simulink model "DTNS_SIM"  (R2022a)
settings: Solver=ode4  StartTime=0.0  StopTime=100  FixedStep=0.01  RelTol=1e-3
PreLoadFcn:
  | listing = dir;
  | if (contains([listing.name], 'MAP')) &&  (contains([listing.name], 'DTNS_SIM.slx'))
  |     addpath('./AGR', './TRN', './TCAF', './FTG', './DYN', './FLCC', './GPS', './RALT', './INS', './MAP');
  |     addpath('./MAP/MAP_DB');
  | else
  |     warning('[DTNS_SIM.slx]는 DTNS 프로젝트 최상단 경로에 위치해야 합니다.');
  | end
  | 
  | load('BUS_STRUCTURE_DYN.mat');
  | load('BUS_STRUCTURE_FLCC.mat');
  | load('BUS_STRUCTURE_RALT.mat');
  | load('BUS_STRUCTURE_INS.mat');
  | load('BUS_STRUCTURE_GPS.mat');
  | load('BusStructureTRN.mat');
  | load('BusStructureLOSR.mat');
  | load('BusStructureHR.mat');
  | load('BusStructureCR.mat');
  | FTG_initState;
InitFcn:
  | listing = dir;
  | if (contains([listing.name], 'MAP')) &&  (contains([listing.name], 'DTNS_SIM.slx'))
  |     addpath('./AGR', './TRN', './TCAF', './FTG', './DYN', './FLCC', './GPS', './RALT', './INS', './MAP');
  |     addpath('./MAP/MAP_DB');
  | else
  |     warning('[DTNS_SIM.slx]는 DTNS 프로젝트 최상단 경로에 위치해야 합니다.');
  | end
  | 
  | load('BUS_STRUCTURE_DYN.mat');
  | load('BUS_STRUCTURE_FLCC.mat');
  | load('BUS_STRUCTURE_RALT.mat');
  | load('BUS_STRUCTURE_INS.mat');
  | load('BUS_STRUCTURE_GPS.mat');
  | load('BusStructureTRN.mat');
  | load('BusStructureLOSR.mat');
  | load('BusStructureHR.mat');
  | load('BusStructureCR.mat');
  | FTG_initState;
undefined symbols (not defined in the file or in its folder): initState
libraries: aerolibconvert2 x16, simulink_extras x5
(part 1 of 2)
settings Model: PacingRate=3  Creator=ASCL  LastModifiedBy=ASCL
settings SolverCC: PositivePriorityOrder=on  AutoInsertRateTranBlk=on
settings DataIOCC: ExternalInput=FTGScenario.getElement('IN_STICK'), [], [], FTGScenario.getElement('IN_FLIGHT_CMD'), []  LoadExternalInput=on  SaveOutput=off  DSMLogging=off  ReturnWorkspaceOutputs=off
settings OptimizationCC: BlockReduction=off  DefaultParameterBehavior=Inlined  UseDivisionForNetSlopeComputation=on  GainParamInheritBuiltInType=on  UseFloatMulNetSlope=on  ExpressionFolding=off  PassReuseOutputArgsAs=Individual arguments  ZeroExternalMemoryAtStartup=off  ZeroInternalMemoryAtStartup=off  EfficientFloat2IntCast=on  LifeSpan=inf  OptimizeBlockOrder=speed  DifferentSizesBufferReuse=on  EfficientTunableParamExpr=on
settings DebuggingCC: SignalInfNanChecking=warning  ReadBeforeWriteMsg=EnableAllAsError  WriteAfterWriteMsg=EnableAllAsError  WriteAfterReadMsg=EnableAllAsError  IntegerOverflowMsg=error  ParameterTunabilityLossMsg=error  UniqueDataStoreMsg=error  AssertControl=DisableAll  NonBusSignalsTreatedAsBus=error  SFInvalidInputDataAccessInChartInitDiag=error  SFTransitionOutsideNaturalParentDiag=error  SFUnreachableExecutionPathDiag=error  SFUndirectedBroadcastEventsDiag=error  IntegerSaturationMsg=error
settings HardwareCC: ProdBitPerPointer=32  ProdBitPerSizeT=32  ProdBitPerPtrDiffT=32  ProdLargestAtomicInteger=Long  ProdLargestAtomicFloat=Double  ProdEndianess=BigEndian  ProdWordSize=32  ProdLongLongMode=on  ProdHWDeviceType=Freescale->MPC83xx
settings ModelReferenceCC: ModelReferenceNumInstancesAllowed=Single
settings SFSimCC: SimCustomHeaderCode="#include \"MAP.h\""  SimUserSources=MAP.c  SimUserLibraries=WS2_32.LIB  CompileTimeRecursionLimit=0  EnableRuntimeRecursion=off  MATLABDynamicMemAlloc=off  CustomCodeGlobalsAsFunctionIO=on
settings RTWCC: SystemTargetFile=ert.tlc  TemplateMakefile=ert_default_tmf  GenerateReport=on  RTWUseSimCustomCode=on  CustomHeaderCode="#include \"MAP.h\""  CustomSource=MAP.c  CustomLibrary=WS2_32.LIB  BuildConfiguration=Faster Runs  IncludeHyperlinkInReport=on  LaunchReport=on  GenerateTraceInfo=on  GenerateTraceReport=on  GenerateTraceReportSl=on  GenerateTraceReportSf=on  GenerateTraceReportEml=on  GenerateCodeMetricsReport=on
settings CodeAppCC: ForceParamTrailComments=on  IgnoreCustomStorageClasses=off  OperatorAnnotations=on  SimulinkDataObjDesc=on  SFDataObjDesc=on  MATLABFcnDesc=on  InsertBlockDesc=on  StateflowObjectComments=on  MATLABSourceComments=on  EnableCustomComments=on  InlinedPrmAccess=Macros  ReqsInCode=on
settings ERTTargetCC: TargetLangStandard=C99 (ISO)  UtilityFuncGeneration=Shared location  GenerateSampleERTMain=on  CombineSignalStateStructs=on  SuppressErrorStatus=on  SupportNonFinite=off  SupportVariableSizeSignals=on  ParenthesesLevel=Standards  CastingMode=Standards  GenerateSharedConstants=off  InlinedParameterPlacement=NonHierarchical  ERTCustomFileTemplate=example_file_process.tlc  RateTransitionBlockCode=Function  PreserveIfCondition=on  ConvertIfToSwitch=off  EnableSignedLeftShifts=off  EnableSignedRightShifts=off

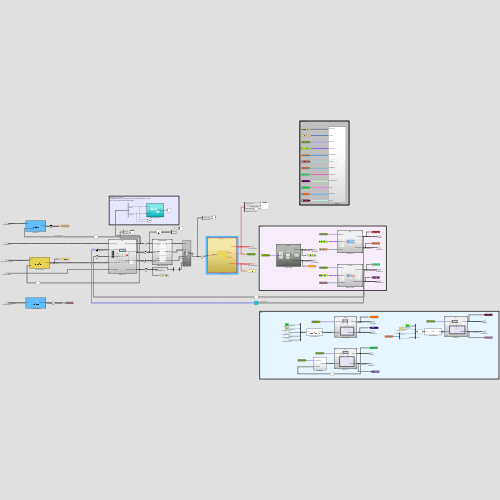
[thumbnail: Simulink's stored preview of the top-level diagram]
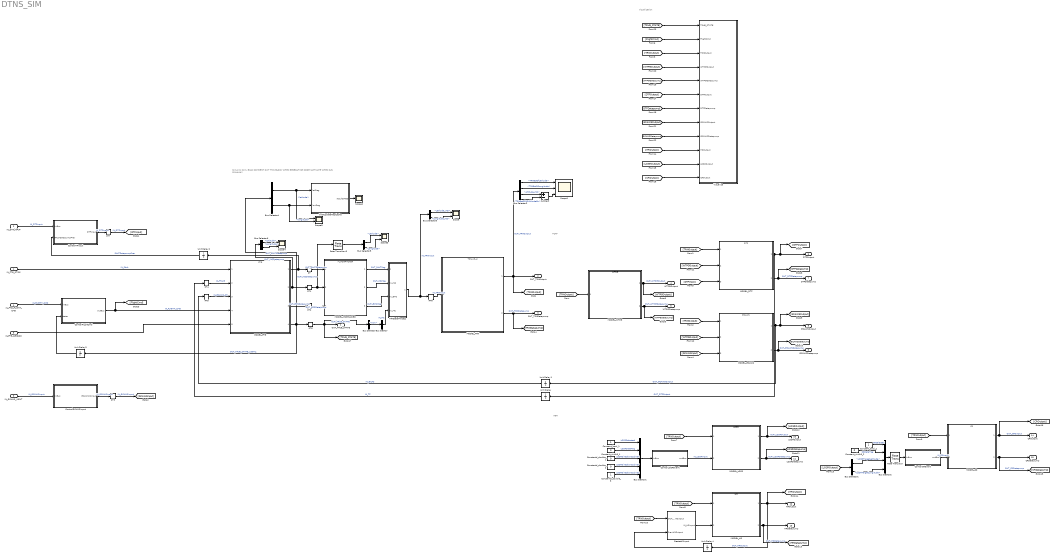
== system DTNS_SIM ==
  note: AGR
  note: TCAF
  note: Visualization
  note: Simulink Only Block
      | COMMENT OUT THIS BLOCK WHEN GENERATING CODE
      | (ACTIVATE WHEN RUN SIMULINK)
  IN_FTG_STICK : Inport  OutDataTypeStr=Bus: BUS_FLCC_STICK  SampleTime=0.01  Interpolate=off  BusOutputAsStruct=on
  IN_DTF_INPUT : Inport  Port=2  OutDataTypeStr=Bus: DTFInput  SampleTime=0.01  Interpolate=off  BusOutputAsStruct=on
  IN_GCAWS_INPUT : Inport  Port=3  OutDataTypeStr=Bus: GCAWSInput  SampleTime=0.01  Interpolate=off  BusOutputAsStruct=on
  IN_FTG_FLIGHT_CMD : Inport  Port=4  OutDataTypeStr=Bus: BUS_FLCC_FLIGHT_CMD  SampleTime=0.01  Interpolate=off  BusOutputAsStruct=on
  IN_FTG_SENSOR : Inport  Port=5  OutDataTypeStr=Bus: BUS_SENSOR_ALL_INPUTSTATUS  SampleTime=0.01  Interpolate=off  BusOutputAsStruct=on
  Bus Creator : BusCreator  Inputs=1  OutDataTypeStr=Bus: TRN_MC  NonVirtualBus=on
      settings: InheritFromInputs=off
  Bus Creator1 : BusCreator  Inputs=5  OutDataTypeStr=Bus: LOSRInput  NonVirtualBus=on
      settings: InheritFromInputs=off
  Bus Creator2 : BusCreator  Inputs=4  OutDataTypeStr=Bus: CRInput
      settings: InheritFromInputs=off
  Bus Selector : BusSelector  OutputSignals=wow
  Bus Selector1 : BusSelector  OutputSignals=LOSRTargetLatitude,LOSRTargetLongitude
  Bus Selector2 : BusSelector  OutputSignals=TRNEstOfLatitude,TRNEstOfLongitude,Altitude_INS,TRNEstOfINSAltitudeErr
  Bus Selector3 : BusSelector  OutputSignals=Latitude_INS,Longitude_INS
  Bus Selector4 : BusSelector  OutputSignals=latitude,longitude
  Bus Selector5 : BusSelector  OutputSignals=Latitude,Longitude
  Bus Selector6 : BusSelector  OutputSignals=Latitude,Longitude
  Constant_bool_1 : Constant  OutDataTypeStr=boolean  SampleTime=0.04
  Constant_bool_2 : Constant  OutDataTypeStr=boolean  SampleTime=0.04
  Constant_uint16_1 : Constant  Value=0  OutDataTypeStr=uint16  SampleTime=0.04
  Constant_uint16_2 : Constant  Value=0  OutDataTypeStr=uint16  SampleTime=0.04
  Constantd_double_1 : Constant  Value=0  OutDataTypeStr=double  SampleTime=0.04
  Constantd_double_2 : Constant  Value=0  OutDataTypeStr=double  SampleTime=0.04
  Constantd_double_3 : Constant  OutDataTypeStr=double  SampleTime=0.04
  ControlCREvent : MATLAB Function  TreatAsAtomicUnit=on  SystemSampleTime=0.04
  ControlFlightCmd : MATLAB Function  TreatAsAtomicUnit=on
  ControlGCAWSInput : MATLAB Function  TreatAsAtomicUnit=on
  ControlLOSREvent : MATLAB Function  TreatAsAtomicUnit=on  SystemSampleTime=0.04
  ControlTFInput : MATLAB Function  TreatAsAtomicUnit=on
  CreateHRInput : Subsystem  TreatAsAtomicUnit=on  PartitionName=CreateHRInput
      settings: RTWSystemCode=Nonreusable function
  InitNUpdateMapCache : Subsystem  TreatAsAtomicUnit=on  PartitionName=InitNUpdateMapCache
  MODEL_CR : ModelReference  ModelNameDialog=CR.slx  SimulationMode=Normal  ScheduleRatesWith=Schedule Editor  ModelReferenceVersion=1.263
  MODEL_DTF : ModelReference  ModelNameDialog=DTF.slx  SimulationMode=Normal  ScheduleRatesWith=Schedule Editor  ModelReferenceVersion=1.443
  MODEL_FTG : ModelReference  ModelNameDialog=FTG.slx  SimulationMode=Normal  ScheduleRatesWith=Schedule Editor  ModelReferenceVersion=1.714
  MODEL_GCAWS : ModelReference  ModelNameDialog=GCAWS.slx  SimulationMode=Normal  ScheduleRatesWith=Schedule Editor  ModelReferenceVersion=1.800
  MODEL_HR : ModelReference  ModelNameDialog=HR.slx  SimulationMode=Normal  ScheduleRatesWith=Schedule Editor  ModelReferenceVersion=1.389
  MODEL_LOSR : ModelReference  ModelNameDialog=LOSR.slx  SimulationMode=Normal  ScheduleRatesWith=Schedule Editor  ModelReferenceVersion=1.371
  MODEL_MSGPACKER : ModelReference  ModelNameDialog=M_MSGPACKER.slx  SimulationMode=Normal  ScheduleRatesWith=Schedule Editor  ModelReferenceVersion=1.319
  MODEL_TRN : ModelReference  ModelNameDialog=TRN_V3_2.slx  SimulationMode=Normal  ScheduleRatesWith=Schedule Editor  CachedPortDiscreteRates=[0.04]  ModelReferenceVersion=2.356
  MODEL_WTPG : ModelReference  ModelNameDialog=WTPG.slx  SimulationMode=Normal  ScheduleRatesWith=Schedule Editor  ModelReferenceVersion=1.459
  RT{,1..3,6..7} (6 alike) : RateTransition  OutPortSampleTime=0.04
  RT4 : RateTransition  OutPortSampleTime=0.01
  RT5 : RateTransition  OutPortSampleTime=0.01
  RT8 : RateTransition
  Rate Transition : RateTransition  OutPortSampleTime=0.04
  Rate Transition3 : RateTransition
  Scope{,3..5} (4 alike) : Scope  NumInputPorts=2
  Scope1 : Scope  NumInputPorts=3
  Scope2 : Scope
  Subtract : Sum  Inputs=+-
  TRNDataProcess : Subsystem  TreatAsAtomicUnit=on  PartitionName=TRNDataProcess
  Unit Delay{,1..2,4} (4 alike) : UnitDelay  SampleTime=-1  HasFrameUpgradeWarning=on
  Unit Delay3 : UnitDelay  InitialCondition=initState  SampleTime=0.01  HasFrameUpgradeWarning=on
  Visualize : Subsystem
  OUT_TRUE_STATE : Outport  OutDataTypeStr=Bus: BUS_DYN_STATE  BusOutputAsStruct=on
  OUT_TRNOutput : Outport  Port=2  OutDataTypeStr=Bus: TRNOutput
  OUT_TRNDatapump : Outport  Port=3  OutDataTypeStr=Bus: TRNDatapump
  WTPGOutput : Outport  Port=4  OutDataTypeStr=Bus: WTPGOutput
  WTPGDatapump : Outport  Port=5  OutDataTypeStr=Bus: WTPGDatapump
  DTFOutput : Outport  Port=6  OutDataTypeStr=Bus: DTFOutput
  DTFDatapump : Outport  Port=7  OutDataTypeStr=Bus: DTFDatapump
  GCAWSOutput : Outport  Port=8  OutDataTypeStr=Bus: GCAWSOutput
  GCAWSDatapump : Outport  Port=9  OutDataTypeStr=Bus: GCAWSDatapump
  LOSROutput : Outport  Port=10  OutDataTypeStr=Bus: LOSROutput  BusOutputAsStruct=on
  LOSRDatapump : Outport  Port=11  OutDataTypeStr=Bus: LOSRDatapump  BusOutputAsStruct=on
  HROutput : Outport  Port=12  OutDataTypeStr=Bus: HROutput  BusOutputAsStruct=on
  HRDatapump : Outport  Port=13  OutDataTypeStr=Bus: HRDatapump  BusOutputAsStruct=on
  CROutput : Outport  Port=14  OutDataTypeStr=Bus: CROutput  BusOutputAsStruct=on
  CRDatapump : Outport  Port=15  OutDataTypeStr=Bus: CRDatapump  BusOutputAsStruct=on
  wires:
  Bus Creator/1 -> TRNDataProcess/4(In_MC)  "IN_MC"
  MODEL_FTG/3 -> RT2/1  "OUT_GPSDatapump"
  MODEL_WTPG/2 -> [WTPGDatapump], WTPGDatapump/1  "OUT_WTPGDatapump"
  MODEL_GCAWS/2 -> [GCAWSDatapump], GCAWSDatapump/1  "OUT_GCAWSDatapump"
  MODEL_TRN/2 -> [TRNDatapump], OUT_TRNDatapump/1  "OUT_TRNDatapump"
  MODEL_GCAWS/1 -> GCAWSOutput/1, [GCAWSOutput], Unit Delay1/1  "OUT_GCAWSOutput"
  IN_GCAWS_INPUT/1 -> ControlGCAWSInput/1(inBus)  "IN_GCAWSInput"
  IN_FTG_FLIGHT_CMD/1 -> ControlFlightCmd/1(inBus)  "IN_FLIGHT_CMD"
  RT6/1 -> [TRUE_STATE], Bus Selector/1, OUT_TRUE_STATE/1  "OUT_TRUE_STATE"
  MODEL_FTG/2 -> Bus Selector6/1, RT1/1  "OUT_INSDatapump"
  Unit Delay1/1 -> RT5/1  "IN_GCAS"
  Unit Delay/1 -> RT4/1  "IN_TF"
  MODEL_FTG/1 -> RT/1, Unit Delay2/1  "OUT_RALTDatapump"
  IN_FTG_STICK/1 -> MODEL_FTG/1  "IN_Stick"
  MODEL_DTF/1 -> DTFOutput/1, [DTFOutput], Unit Delay/1  "OUT_DTFOutput"
  ControlFlightCmd/1(outBus) -> MODEL_FTG/4, [FlightCmd]  "IN_FLIGHT_CMD"
  IN_DTF_INPUT/1 -> ControlTFInput/1(inBus)  "IN_DTFInput"
  MODEL_MSGPACKER/3 -> TRNDataProcess/3(In_GPS)  "OUT_GPSMsg"
  MODEL_MSGPACKER/1 -> TRNDataProcess/1(In_RALT)  "OUT_RALTMsg"
  MODEL_MSGPACKER/2 -> TRNDataProcess/2(In_INS)  "OUT_INSMsg"
  InitNUpdateMapCache/1(resultDTED) -> Scope2/1
  IN_FTG_SENSOR/1 -> MODEL_FTG/5
  RT7/1 -> [DTFInput]  "IN_DTFInput"
  Unit Delay2/1 -> ControlTFInput/2(RALTDatapumpPrev)  "RALTDatapumpPrev"
  RT3/1 -> [GCAWSInput]  "IN_GCAWSInput"
  Unit Delay3/1 -> ControlFlightCmd/2(state)
  TRNDataProcess/1(TRN INPUT) -> Bus Selector3/1, RT8/1  "IN_TRNInput"
  RT/1 -> MODEL_MSGPACKER/1  "OUT_RALTDatapump"
  RT1/1 -> Rate Transition3/1, MODEL_MSGPACKER/2  "OUT_INSDatapump"
  RT2/1 -> MODEL_MSGPACKER/3  "OUT_GPSDatapump"
  RT4/1 -> MODEL_FTG/2  "IN_TF_25"
  RT5/1 -> MODEL_FTG/3  "IN_GCAWS_25"
  MODEL_FTG/4 -> Unit Delay3/1, Bus Selector4/1, RT6/1  "OUT_TRUE_STATE_100HZ"
  Constant_uint16_2/1 -> Bus Creator2/2  "CRDataTag"
  MODEL_HR/2 -> HRDatapump/1, [HRDatapump]  "OUT_HRDatapump"
  Bus Creator1/1 -> ControlLOSREvent/1(inBus)
  Constant_uint16_1/1 -> Bus Creator1/2  "LOSRDataTag"
  MODEL_LOSR/1 -> LOSROutput/1, [LOSROutput]  "OUT_LOSROutput"
  MODEL_TRN/1 -> Bus Selector2/1, OUT_TRNOutput/1, [TRNOutput]  "OUT_TRNOutput"
  Bus Selector1/1 -> Bus Creator2/3  "<LOSRTargetLatitude>"
  Bus Selector1/2 -> Bus Creator2/4  "<LOSRTargetLongitude>"
  Bus Creator2/1 -> Rate Transition/1
  Constant_bool_2/1 -> Bus Creator2/1  "CRSelected"
  MODEL_CR/2 -> [CRDatapump], CRDatapump/1  "OUT_CRDatapump"
  MODEL_CR/1 -> [CROutput], CROutput/1  "OUT_CROutput"
  Constantd_double_2/1 -> Bus Creator1/4  "LOSRDirectionCosineY"
  Constant_bool_1/1 -> Bus Creator1/1  "LOSRSelected"
  ControlCREvent/1(outBus) -> MODEL_CR/2  "IN_CRInput"
  ControlLOSREvent/1(outBus) -> MODEL_LOSR/2  "IN_LOSRInput"
  Constantd_double_3/1 -> Bus Creator1/5  "LOSRDirectionCosineZ"
  Constantd_double_1/1 -> Bus Creator1/3  "LOSRDirectionCosineX"
  MODEL_LOSR/2 -> [LOSRDatapump], LOSRDatapump/1  "OUT_LOSRDatapump"
  Rate Transition/1 -> ControlCREvent/1(inBus)
  MODEL_DTF/2 -> [DTFDatapump], DTFDatapump/1  "OUT_DTFDatapump"
  Unit Delay4/1 -> CreateHRInput/2(PrevHROutput)
  CreateHRInput/1(IN_HRInput) -> MODEL_HR/2
  MODEL_WTPG/1 -> [WTPGOutput], WTPGOutput/1  "OUT_WTPGOutput"
  [TRNOutput] -> MODEL_WTPG/1
  [GCAWSInput] -> MODEL_GCAWS/3
  [DTFInput] -> MODEL_DTF/3
  [TRNOutput] -> MODEL_CR/1
  MODEL_HR/1 -> HROutput/1, Unit Delay4/1, [HROutput]  "OUT_HROutput"
  [WTPGOutput] -> MODEL_DTF/2
  [WTPGOutput] -> MODEL_GCAWS/2
  [LOSROutput] -> Bus Selector1/1
  [TRNOutput] -> Visualize/3(TRNOutput)
  [FlightCmd] -> Visualize/2(FlightCmd)
  [HROutput] -> Visualize/10(HROutput)
  [LOSROutput] -> Visualize/11(LOSROutput)
  [CROutput] -> Visualize/12(CROutput)
  [TRNOutput] -> MODEL_DTF/1
  [TRNOutput] -> MODEL_GCAWS/1
  [TRNOutput] -> CreateHRInput/1(OUT_TRNOutput)
  [TRNOutput] -> MODEL_HR/1
  [TRNOutput] -> MODEL_LOSR/1
  ControlGCAWSInput/1(GCAWWSInput) -> RT3/1  "IN_GCAWSInput"
  ControlTFInput/1(DTFInput) -> RT7/1  "IN_DTFInput"
  Bus Selector/1 -> Bus Creator/1  "<wow>"
  Bus Selector3/1 -> Scope/1  "<Latitude_INS>"
  Bus Selector3/2 -> Scope/2  "<Longitude_INS>"
  Bus Selector2/1 -> Scope1/1  "<TRNEstOfLatitude>"
  Bus Selector2/2 -> Scope1/2  "<TRNEstOfLongitude>"
  Bus Selector5/1 -> Scope3/1  "<Latitude>"
  Bus Selector5/2 -> Scope3/2  "<Longitude>"
  Rate Transition3/1 -> Bus Selector5/1
  RT8/1 -> MODEL_TRN/1  "IN_TRNInput"
  Bus Selector6/2 -> Scope4/2  "<Longitude>"
  Bus Selector6/1 -> Scope4/1  "<Latitude>"
  Bus Selector4/1 -> Scope5/1, InitNUpdateMapCache/1(latDeg)  "<latitude>"
  Bus Selector4/2 -> Scope5/2, InitNUpdateMapCache/2(lonDeg)  "<longitude>"
  [WTPGOutput] -> Visualize/4(WTPGOutput)
  [WTPGDatapump] -> Visualize/5(WTPGDatapump)
  [DTFOutput] -> Visualize/6(DTFOutput)
  [DTFDatapump] -> Visualize/7(DTFDatapump)
  [GCAWSOutput] -> Visualize/8(GCAWSOutput)
  [GCAWSDatapump] -> Visualize/9(GCAWSDatapump)
  [TRUE_STATE] -> Visualize/1(TRUE_STATE)
  Subtract/1 -> Scope1/3
  Bus Selector2/3 -> Subtract/1  "<Altitude_INS>"
  Bus Selector2/4 -> Subtract/2  "<TRNEstOfINSAltitudeErr>"

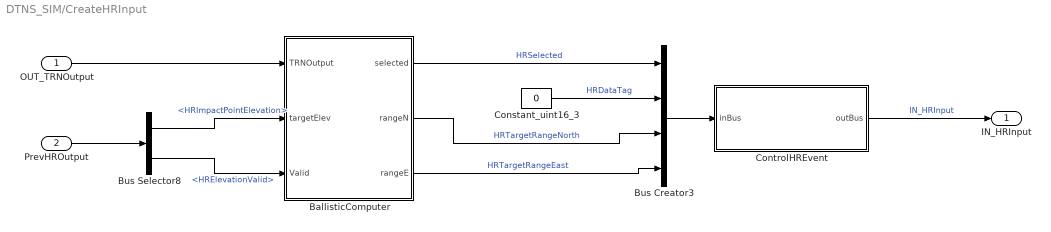
== system DTNS_SIM/CreateHRInput ==
  OUT_TRNOutput : Inport
  PrevHROutput : Inport  Port=2
  BallisticComputer : MATLAB Function  TreatAsAtomicUnit=on  SystemSampleTime=0.04
  Bus Creator3 : BusCreator  Inputs=4  OutDataTypeStr=Bus: HRInput  NonVirtualBus=on
      settings: InheritFromInputs=off
  Bus Selector8 : BusSelector  OutputSignals=HRImpactPointElevation,HRElevationValid
  Constant_uint16_3 : Constant  Value=0  OutDataTypeStr=uint16  SampleTime=0.04
  ControlHREvent : MATLAB Function  TreatAsAtomicUnit=on  SystemSampleTime=0.04
  IN_HRInput : Outport
  wires:
  BallisticComputer/3(rangeE) -> Bus Creator3/4  "HRTargetRangeEast"
  BallisticComputer/2(rangeN) -> Bus Creator3/3  "HRTargetRangeNorth"
  Bus Selector8/1 -> BallisticComputer/2(targetElev)  "<HRImpactPointElevation>"
  BallisticComputer/1(selected) -> Bus Creator3/1  "HRSelected"
  OUT_TRNOutput/1 -> BallisticComputer/1(TRNOutput)
  Constant_uint16_3/1 -> Bus Creator3/2  "HRDataTag"
  Bus Creator3/1 -> ControlHREvent/1(inBus)
  Bus Selector8/2 -> BallisticComputer/3(Valid)  "<HRElevationValid>"
  PrevHROutput/1 -> Bus Selector8/1
  ControlHREvent/1(outBus) -> IN_HRInput/1  "IN_HRInput"

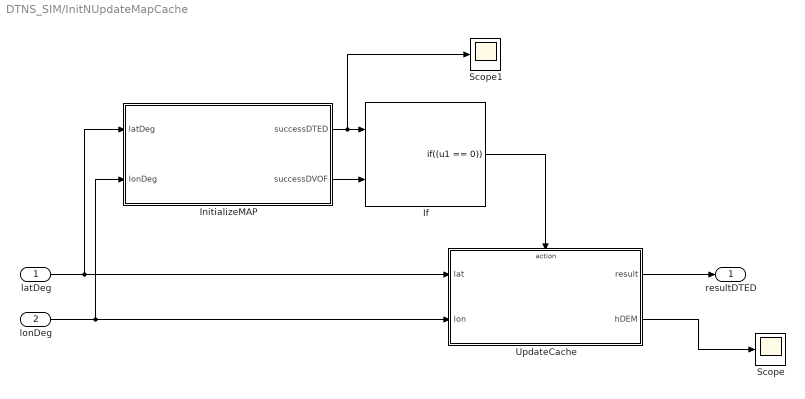
== system DTNS_SIM/InitNUpdateMapCache ==
  latDeg : Inport  OutDataTypeStr=double
  lonDeg : Inport  Port=2  OutDataTypeStr=double
  If : If  NumInputs=2  IfExpression=(u1 == 0)  ShowElse=off
  InitializeMAP : MATLAB Function  TreatAsAtomicUnit=on
  Scope : Scope
  Scope1 : Scope
  UpdateCache : Subsystem  TreatAsAtomicUnit=on
  resultDTED : Outport  VectorParamsAs1DForOutWhenUnconnected=off
  wires:
  lonDeg/1 -> InitializeMAP/2(lonDeg), UpdateCache/2(lon)
  UpdateCache/1(result) -> resultDTED/1
  InitializeMAP/1(successDTED) -> Scope1/1, If/1
  latDeg/1 -> InitializeMAP/1(latDeg), UpdateCache/1(lat)
  InitializeMAP/2(successDVOF) -> If/2
  If/1 -> UpdateCache/Action
  UpdateCache/2(hDEM) -> Scope/1

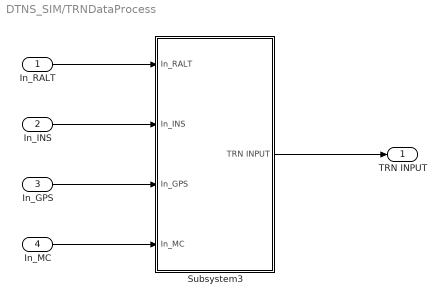
== system DTNS_SIM/TRNDataProcess ==
  In_RALT : Inport
  In_INS : Inport  Port=2
  In_GPS : Inport  Port=3
  In_MC : Inport  Port=4
  Subsystem3 : Subsystem
  TRN INPUT : Outport
  wires:
  In_GPS/1 -> Subsystem3/3(In_GPS)
  In_MC/1 -> Subsystem3/4(In_MC)
  Subsystem3/1(TRN INPUT) -> TRN INPUT/1
  In_RALT/1 -> Subsystem3/1(In_RALT)
  In_INS/1 -> Subsystem3/2(In_INS)

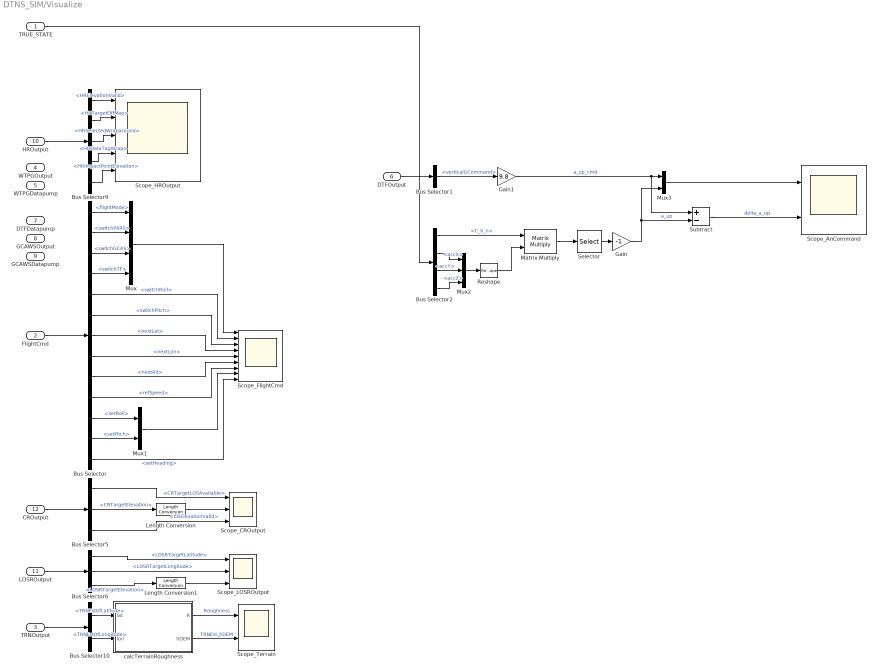
== system DTNS_SIM/Visualize ==
  TRUE_STATE : Inport
  FlightCmd : Inport  Port=2
  TRNOutput : Inport  Port=3
  WTPGOutput : Inport  Port=4
  WTPGDatapump : Inport  Port=5
  DTFOutput : Inport  Port=6
  DTFDatapump : Inport  Port=7
  GCAWSOutput : Inport  Port=8
  GCAWSDatapump : Inport  Port=9
  HROutput : Inport  Port=10
  LOSROutput : Inport  Port=11
  CROutput : Inport  Port=12
  Bus Selector : BusSelector  OutputSignals=flightMode,switchPARS,switchGCAS,switchTF,switchRoll,switchPitch,nextLat,nextLon,nextAlt,refSpeed,setRoll,setPitch,setHeading
  Bus Selector1 : BusSelector  OutputSignals=verticalGCommand
  Bus Selector10 : BusSelector  OutputSignals=TRNEstOfLatitude,TRNEstOfLongitude
  Bus Selector2 : BusSelector  OutputSignals=C_b_n,accX,accY,accZ
  Bus Selector5 : BusSelector  OutputSignals=CRTargetLOSAvailable,CRTargetElevation,CRElevationValid
  Bus Selector6 : BusSelector  OutputSignals=LOSRTargetLatitude,LOSRTargetLongitude,LOSRTargetElevation
  Bus Selector9 : BusSelector  OutputSignals=HRElevationValid,HRTargetOffMap,HRSelectedWraparound,HRDataTagWrap,HRImpactPointElevation
  Gain : Gain  Gain=-1
  Gain1 : Gain  Gain=9.8
  Length Conversion : aerolibconvert2/Length Conversion  IU=ft  OU=m
  Length Conversion1 : aerolibconvert2/Length Conversion  IU=ft  OU=m
  Matrix Multiply : Product  Multiplication=Matrix(*)
  Mux : Mux
  Mux1 : Mux  Inputs=2
  Mux2 : Mux  Inputs=3
  Mux3 : Mux  Inputs=2
  Reshape : Reshape  OutputDimensionality=Column vector (2-D)
  Scope_AnCommand : Scope  NumInputPorts=2
  Scope_CROutput : Scope  NumInputPorts=3
  Scope_FlightCmd : Scope  NumInputPorts=9
  Scope_HROutput : Scope  NumInputPorts=5
  Scope_LOSROutput : Scope  NumInputPorts=3
  Scope_Terrain : Scope  NumInputPorts=2
  Selector : Selector  NumberOfDimensions=2  InputPortWidth=3  IndexOptions=Index vector (dialog),Index vector (dialog)  Indices=[3],1  OutputSizes=1,1
  Subtract : Sum  Inputs=+-
  calcTerrainRoughness : MATLAB Function  TreatAsAtomicUnit=on
  wires:
  calcTerrainRoughness/2(hDEM) -> Scope_Terrain/2  "TRNEst_hDEM"
  FlightCmd/1 -> Bus Selector/1
  HROutput/1 -> Bus Selector9/1
  Bus Selector5/1 -> Scope_CROutput/1  "<CRTargetLOSAvailable>"
  Bus Selector9/5 -> Scope_HROutput/5  "<HRImpactPointElevation>"
  Bus Selector9/3 -> Scope_HROutput/3  "<HRSelectedWraparound>"
  Bus Selector10/1 -> calcTerrainRoughness/1(lat)  "<TRNEstOfLatitude>"
  Bus Selector6/2 -> Scope_LOSROutput/2  "<LOSRTargetLongitude>"
  Bus Selector10/2 -> calcTerrainRoughness/2(lon)  "<TRNEstOfLongitude>"
  Bus Selector5/3 -> Scope_CROutput/3  "<CRElevationValid>"
  Bus Selector5/2 -> Length Conversion/1  "<CRTargetElevation>"
  Bus Selector9/1 -> Scope_HROutput/1  "<HRElevationValid>"
  Bus Selector/6 -> Scope_FlightCmd/3  "<switchPitch>"
  Bus Selector/10 -> Scope_FlightCmd/7  "<refSpeed>"
  Bus Selector9/4 -> Scope_HROutput/4  "<HRDataTagWrap>"
  Bus Selector/7 -> Scope_FlightCmd/4  "<nextLat>"
  TRNOutput/1 -> Bus Selector10/1
  Bus Selector6/1 -> Scope_LOSROutput/1  "<LOSRTargetLatitude>"
  Bus Selector/11 -> Mux1/1  "<setRoll>"
  Mux/1 -> Scope_FlightCmd/1
  Bus Selector/12 -> Mux1/2  "<setPitch>"
  Bus Selector/8 -> Scope_FlightCmd/5  "<nextLon>"
  Bus Selector/4 -> Mux/4  "<switchTF>"
  Bus Selector/13 -> Scope_FlightCmd/9  "<setHeading>"
  Bus Selector/9 -> Scope_FlightCmd/6  "<nextAlt>"
  Bus Selector/5 -> Scope_FlightCmd/2  "<switchRoll>"
  Bus Selector9/2 -> Scope_HROutput/2  "<HRTargetOffMap>"
  Bus Selector/1 -> Mux/1  "<flightMode>"
  CROutput/1 -> Bus Selector5/1
  Bus Selector/2 -> Mux/2  "<switchPARS>"
  Mux1/1 -> Scope_FlightCmd/8
  Bus Selector/3 -> Mux/3  "<switchGCAS>"
  LOSROutput/1 -> Bus Selector6/1
  calcTerrainRoughness/1(R) -> Scope_Terrain/1  "Roughness"
  Length Conversion/1 -> Scope_CROutput/2
  Bus Selector6/3 -> Length Conversion1/1  "<LOSRTargetElevation>"
  Length Conversion1/1 -> Scope_LOSROutput/3
  DTFOutput/1 -> Bus Selector1/1
  Bus Selector1/1 -> Gain1/1  "<verticalGCommand>"
  TRUE_STATE/1 -> Bus Selector2/1
  Mux2/1 -> Reshape/1
  Bus Selector2/3 -> Mux2/2  "<accY>"
  Bus Selector2/2 -> Mux2/1  "<accX>"
  Bus Selector2/4 -> Mux2/3  "<accZ>"
  Bus Selector2/1 -> Matrix Multiply/1  "<C_b_n>"
  Reshape/1 -> Matrix Multiply/2
  Matrix Multiply/1 -> Selector/1
  Gain/1 -> Mux3/2, Subtract/2  "a_up"
  Mux3/1 -> Scope_AnCommand/1
  Selector/1 -> Gain/1
  Subtract/1 -> Scope_AnCommand/2  "delta_a_up"
  Gain1/1 -> Subtract/1, Mux3/1  "a_up_cmd"

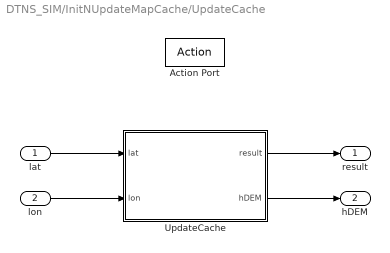
== system DTNS_SIM/InitNUpdateMapCache/UpdateCache ==
  lat : Inport
  lon : Inport  Port=2
  Action Port : ActionPort  ActionPortLabel=if((u1 == 0))
  UpdateCache : MATLAB Function  TreatAsAtomicUnit=on
  result : Outport  VectorParamsAs1DForOutWhenUnconnected=off
  hDEM : Outport  Port=2
  wires:
  UpdateCache/1(result) -> result/1
  lat/1 -> UpdateCache/1(lat)
  lon/1 -> UpdateCache/2(lon)
  UpdateCache/2(hDEM) -> hDEM/1

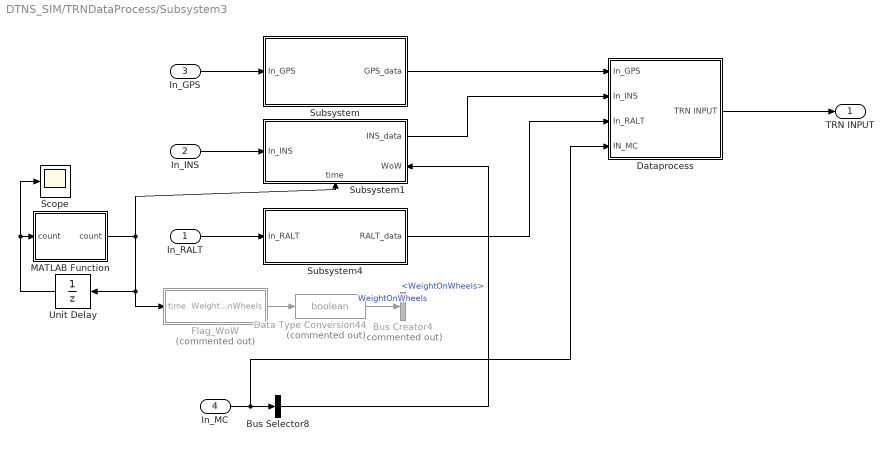
== system DTNS_SIM/TRNDataProcess/Subsystem3 ==
  In_RALT : Inport
  In_INS : Inport  Port=2
  In_GPS : Inport  Port=3
  In_MC : Inport  Port=4
  Bus Creator4 : BusCreator  Commented=on  Inputs=1  OutDataTypeStr=Bus: TRN_MC  NonVirtualBus=on
      settings: InheritFromInputs=off
  Bus Selector8 : BusSelector  OutputSignals=WeightOnWheels
  Data Type Conversion44 : DataTypeConversion  Commented=on  OutDataTypeStr=boolean  SaturateOnIntegerOverflow=off  RndMeth=Floor
  Dataprocess : Subsystem
  Flag_WoW : MATLAB Function  Commented=on  TreatAsAtomicUnit=on
  MATLAB Function : MATLAB Function  TreatAsAtomicUnit=on
  Scope : Scope
  Subsystem : Subsystem
  Subsystem1 : Subsystem
      settings: PortSchema="{\"entries\":[{\"content\":{\"sides\":[{\"content\":{\"connectorIds\":[\"In1\"]},\"type\":\"ConnectorPlacement.EquallySpacedRectSide\",\"uuid\":\"627687e9-0c69-45fe-ab30-f2b8c78c94c9\"},{\"content\":{\"connectorIds\":[\"Out1\",\"In3\"],\"side\":\"RIGHT\"},\"type\":\"ConnectorPlacement.EquallySpacedRectSide\",\"uuid\":\"cca5eff4-b683-4134-86dd-9b38fc1aef42\"},{\"content\":{\"connectorIds\":[],\"side\":\"TOP\"},\"type\":\"ConnectorPlacement.EquallySpacedRectSide\",\"uuid\":\"db09404b-1405-40a7-9047-09d57f6d1ee9\"},{\"content\":{\"connectorIds\":[\"In2\"],\"side\":\"BOTTOM\"},\"type\":\"ConnectorPlacement.EquallySpacedRectSide\",\"uuid\":\"43181e0c-7a64-4398-bddd-a3419aca840e\"}]},\"type\":\"ConnectorPlacement.EquallySpacedConnector\",\"uuid\":\"8e5a566a-2f6b-4dcc-950b-8518900682ca\"}],\"packageUris\":[\"http://schema.mathworks.com/mf0/Connector/R2020b\"],\"version\":\"1.0\"}"
  Subsystem4 : Subsystem
  Unit Delay : UnitDelay  SampleTime=-1  HasFrameUpgradeWarning=on
  TRN INPUT : Outport
  wires:
  Flag_WoW/1(WeightOnWheels) -> Data Type Conversion44/1
  Data Type Conversion44/1 -> Bus Creator4/1  "WeightOnWheels"
  Subsystem1/1(INS_data) -> Dataprocess/2(In_INS)
  Subsystem/1(GPS_data) -> Dataprocess/1(In_GPS)
  Dataprocess/1(TRN INPUT) -> TRN INPUT/1
  In_MC/1 -> Dataprocess/4(IN_MC), Bus Selector8/1
  In_GPS/1 -> Subsystem/1(In_GPS)
  In_INS/1 -> Subsystem1/1(In_INS)
  In_RALT/1 -> Subsystem4/1(In_RALT)
  Subsystem4/1(RALT_data) -> Dataprocess/3(In_RALT)
  MATLAB Function/1(count) -> Unit Delay/1, Flag_WoW/1(time), Subsystem1/2(time)
  Unit Delay/1 -> Scope/1, MATLAB Function/1("count ")
  Bus Selector8/1 -> Subsystem1/3(WoW)  "<WeightOnWheels>"

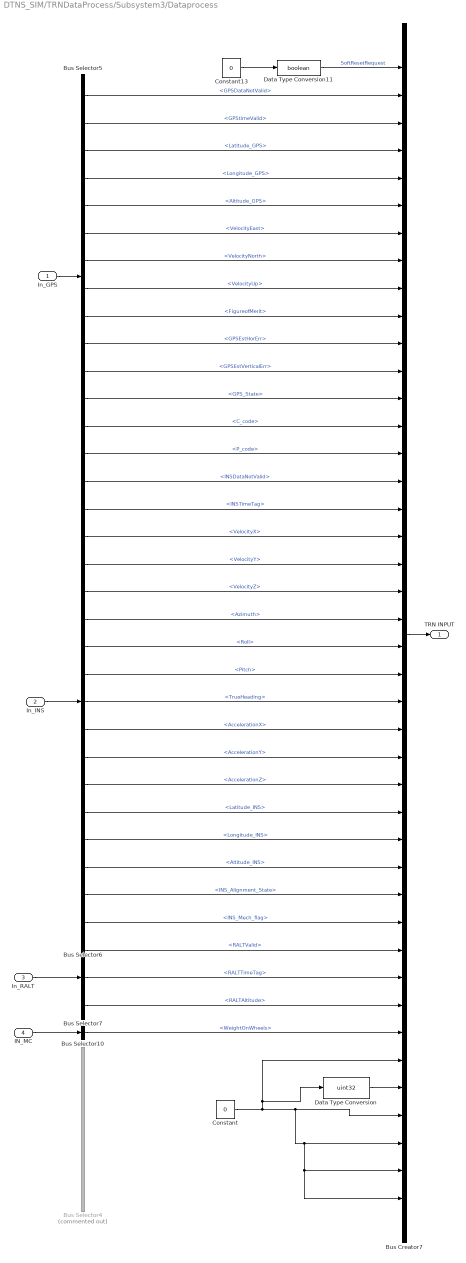
== system DTNS_SIM/TRNDataProcess/Subsystem3/Dataprocess ==
  In_GPS : Inport
  In_INS : Inport  Port=2
  In_RALT : Inport  Port=3
  IN_MC : Inport  Port=4
  Bus Creator7 : BusCreator  Inputs=42  OutDataTypeStr=Bus: TRNInput  NonVirtualBus=on
      settings: InheritFromInputs=off
  Bus Selector10 : BusSelector  OutputSignals=WeightOnWheels
  Bus Selector4 : BusSelector  Commented=on  OutputSignals=MAP_hight,Map_Level,Map_size,Map_resolution,bottomLat,leftLon
  Bus Selector5 : BusSelector  OutputSignals=GPSDataNotValid,GPStimeValid,Latitude_GPS,Longitude_GPS,Altitude_GPS,VelocityEast,VelocityNorth,VelocityUp,FigureofMerit,GPSEstHorErr,GPSEstVerticalErr,GPS_State,C_code,P_code
  Bus Selector6 : BusSelector  OutputSignals=INSDataNotValid,INSTimeTag,VelocityX,VelocityY,VelocityZ,Azimuth,Roll,Pitch,TrueHeading,AccelerationX,AccelerationY,AccelerationZ,Latitude_INS,Longitude_INS,Altitude_INS,INS_Alignment_State,INS_Mech_flag
  Bus Selector7 : BusSelector  OutputSignals=RALTValid,RALTTimeTag,RALTAltitude
  Constant : Constant  Value=0
  Constant13 : Constant  Value=0
  Data Type Conversion : DataTypeConversion  OutDataTypeStr=uint32  SaturateOnIntegerOverflow=off  RndMeth=Floor
  Data Type Conversion11 : DataTypeConversion  OutDataTypeStr=boolean  SaturateOnIntegerOverflow=off  RndMeth=Floor
  TRN INPUT : Outport  OutDataTypeStr=Bus: TRNInput  VectorParamsAs1DForOutWhenUnconnected=off
  wires:
  Bus Selector5/8 -> Bus Creator7/9  "<VelocityUp>"
  Bus Selector6/16 -> Bus Creator7/31  "<INS_Alignment_State>"
  Bus Selector5/7 -> Bus Creator7/8  "<VelocityNorth>"
  In_GPS/1 -> Bus Selector5/1
  Bus Selector5/4 -> Bus Creator7/5  "<Longitude_GPS>"
  Bus Selector5/11 -> Bus Creator7/12  "<GPSEstVerticalErr>"
  Bus Selector5/3 -> Bus Creator7/4  "<Latitude_GPS>"
  Bus Selector6/13 -> Bus Creator7/28  "<Latitude_INS>"
  Bus Selector6/14 -> Bus Creator7/29  "<Longitude_INS>"
  Bus Selector5/12 -> Bus Creator7/13  "<GPS_State>"
  Bus Selector6/9 -> Bus Creator7/24  "<TrueHeading>"
  Bus Selector5/14 -> Bus Creator7/15  "<P_code>"
  Bus Selector6/1 -> Bus Creator7/16  "<INSDataNotValid>"
  Bus Creator7/1 -> TRN INPUT/1
  Data Type Conversion11/1 -> Bus Creator7/1  "SoftResetRequest"
  Bus Selector5/6 -> Bus Creator7/7  "<VelocityEast>"
  Bus Selector6/12 -> Bus Creator7/27  "<AccelerationZ>"
  Bus Selector6/3 -> Bus Creator7/18  "<VelocityX>"
  Bus Selector5/13 -> Bus Creator7/14  "<C_code>"
  Bus Selector6/6 -> Bus Creator7/21  "<Azimuth>"
  Bus Selector5/5 -> Bus Creator7/6  "<Altitude_GPS>"
  Bus Selector6/10 -> Bus Creator7/25  "<AccelerationX>"
  Bus Selector7/3 -> Bus Creator7/35  "<RALTAltitude>"
  In_INS/1 -> Bus Selector6/1
  Bus Selector7/1 -> Bus Creator7/33  "<RALTValid>"
  Bus Selector5/1 -> Bus Creator7/2  "<GPSDataNotValid>"
  Bus Selector10/1 -> Bus Creator7/36  "<WeightOnWheels>"
  Bus Selector6/17 -> Bus Creator7/32  "<INS_Mech_flag>"
  Bus Selector6/4 -> Bus Creator7/19  "<VelocityY>"
  Bus Selector6/7 -> Bus Creator7/22  "<Roll>"
  Constant13/1 -> Data Type Conversion11/1
  Bus Selector7/2 -> Bus Creator7/34  "<RALTTimeTag>"
  Bus Selector6/5 -> Bus Creator7/20  "<VelocityZ>"
  Bus Selector6/2 -> Bus Creator7/17  "<INSTimeTag>"
  Bus Selector6/8 -> Bus Creator7/23  "<Pitch>"
  Bus Selector5/2 -> Bus Creator7/3  "<GPStimeValid>"
  Bus Selector5/10 -> Bus Creator7/11  "<GPSEstHorErr>"
  Bus Selector6/15 -> Bus Creator7/30  "<Altitude_INS>"
  Bus Selector6/11 -> Bus Creator7/26  "<AccelerationY>"
  Bus Selector5/9 -> Bus Creator7/10  "<FigureofMerit>"
  In_RALT/1 -> Bus Selector7/1
  IN_MC/1 -> Bus Selector10/1
  Constant/1 -> Bus Creator7/39, Bus Creator7/40, Bus Creator7/42, Bus Creator7/41, Bus Creator7/37, Data Type Conversion/1
  Data Type Conversion/1 -> Bus Creator7/38

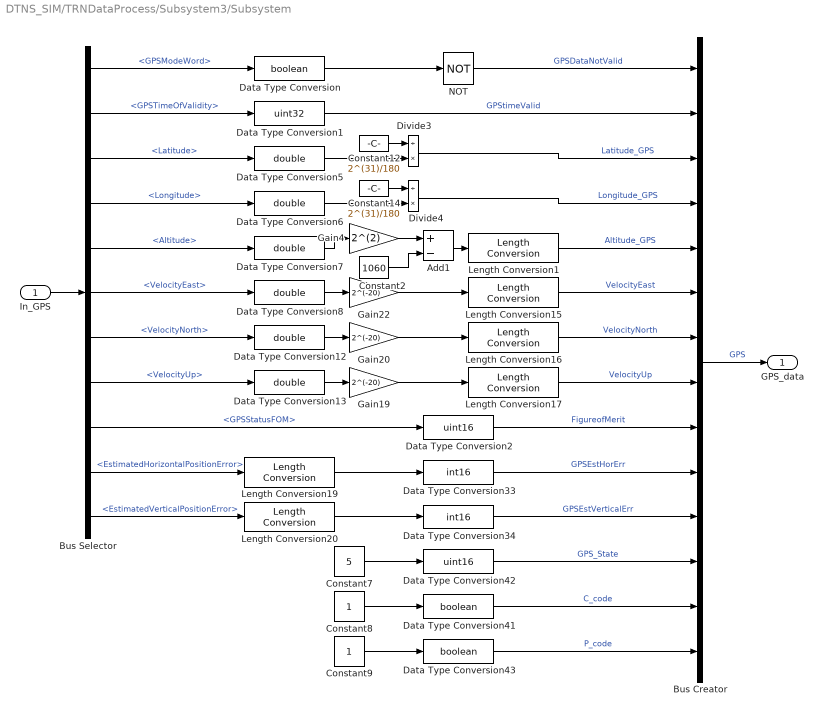
== system DTNS_SIM/TRNDataProcess/Subsystem3/Subsystem ==
  In_GPS : Inport
  Add1 : Sum  Inputs=+-
  Bus Creator : BusCreator  Inputs=14  OutDataTypeStr=Bus: TRN_GPS  NonVirtualBus=on
      settings: InheritFromInputs=off
  Bus Selector : BusSelector  OutputSignals=GPSModeWord,GPSTimeOfValidity,Latitude,Longitude,Altitude,VelocityEast,VelocityNorth,VelocityUp,GPSStatusFOM,EstimatedHorizontalPositionError,EstimatedVerticalPositionError
  Constant12 : Constant  Value=2^(31)/180
  Constant14 : Constant  Value=2^(31)/180
  Constant2 : Constant  Value=1060
  Constant7 : Constant  Value=5
  Constant8 : Constant
  Constant9 : Constant
  Data Type Conversion : DataTypeConversion  OutDataTypeStr=boolean  SaturateOnIntegerOverflow=off  RndMeth=Floor
  Data Type Conversion1 : DataTypeConversion  OutDataTypeStr=uint32  SaturateOnIntegerOverflow=off  RndMeth=Floor
  Data Type Conversion{5..8,12..13} (6 alike) : DataTypeConversion  OutDataTypeStr=double  SaturateOnIntegerOverflow=off  RndMeth=Floor
  Data Type Conversion2 : DataTypeConversion  OutDataTypeStr=uint16  SaturateOnIntegerOverflow=off  RndMeth=Floor
  Data Type Conversion33 : DataTypeConversion  OutDataTypeStr=int16  SaturateOnIntegerOverflow=off  RndMeth=Floor
  Data Type Conversion34 : DataTypeConversion  OutDataTypeStr=int16  SaturateOnIntegerOverflow=off  RndMeth=Floor
  Data Type Conversion41 : DataTypeConversion  OutDataTypeStr=boolean  SaturateOnIntegerOverflow=off  RndMeth=Floor
  Data Type Conversion42 : DataTypeConversion  OutDataTypeStr=uint16  SaturateOnIntegerOverflow=off  RndMeth=Floor
  Data Type Conversion43 : DataTypeConversion  OutDataTypeStr=boolean  SaturateOnIntegerOverflow=off  RndMeth=Floor
  Divide3 : Product  Inputs=/*
  Divide4 : Product  Inputs=/*
  Gain19 : Gain  Gain=2^(-20)
  Gain20 : Gain  Gain=2^(-20)
  Gain22 : Gain  Gain=2^(-20)
  Gain4 : Gain  Gain=2^(2)
  Length Conversion{1,15..17,19..20} (6 alike) : aerolibconvert2/Length Conversion  IU=ft  OU=m
  NOT : Logic  Operator=NOT  IconShape=distinctive  AllPortsSameDT=off  OutDataTypeStr=boolean
  GPS_data : Outport
  wires:
  Length Conversion1/1 -> Bus Creator/5  "Altitude_GPS"
  Bus Selector/7 -> Data Type Conversion12/1  "<VelocityNorth>"
  Bus Selector/2 -> Data Type Conversion1/1  "<GPSTimeOfValidity>"
  Bus Selector/3 -> Data Type Conversion5/1  "<Latitude>"
  Gain4/1 -> Add1/1
  Data Type Conversion33/1 -> Bus Creator/10  "GPSEstHorErr"
  Bus Selector/5 -> Data Type Conversion7/1  "<Altitude>"
  Data Type Conversion8/1 -> Gain22/1
  Data Type Conversion41/1 -> Bus Creator/13  "C_code"
  Bus Selector/11 -> Length Conversion20/1  "<EstimatedVerticalPositionError>"
  Gain20/1 -> Length Conversion16/1
  Bus Selector/10 -> Length Conversion19/1  "<EstimatedHorizontalPositionError>"
  Divide3/1 -> Bus Creator/3  "Latitude_GPS"
  Bus Selector/6 -> Data Type Conversion8/1  "<VelocityEast>"
  Data Type Conversion13/1 -> Gain19/1
  Data Type Conversion6/1 -> Divide4/2
  Data Type Conversion34/1 -> Bus Creator/11  "GPSEstVerticalErr"
  Data Type Conversion42/1 -> Bus Creator/12  "GPS_State"
  Gain22/1 -> Length Conversion15/1
  Length Conversion20/1 -> Data Type Conversion34/1
  Data Type Conversion5/1 -> Divide3/2
  Add1/1 -> Length Conversion1/1
  Data Type Conversion1/1 -> Bus Creator/2  "GPStimeValid"
  Gain19/1 -> Length Conversion17/1
  Constant8/1 -> Data Type Conversion41/1
  Data Type Conversion2/1 -> Bus Creator/9  "FigureofMerit"
  Data Type Conversion7/1 -> Gain4/1
  Bus Selector/8 -> Data Type Conversion13/1  "<VelocityUp>"
  Constant7/1 -> Data Type Conversion42/1
  Bus Selector/4 -> Data Type Conversion6/1  "<Longitude>"
  Bus Selector/9 -> Data Type Conversion2/1  "<GPSStatusFOM>"
  Length Conversion17/1 -> Bus Creator/8  "VelocityUp"
  Length Conversion16/1 -> Bus Creator/7  "VelocityNorth"
  Bus Creator/1 -> GPS_data/1  "GPS"
  Data Type Conversion12/1 -> Gain20/1
  Constant2/1 -> Add1/2
  Length Conversion15/1 -> Bus Creator/6  "VelocityEast"
  Length Conversion19/1 -> Data Type Conversion33/1
  Divide4/1 -> Bus Creator/4  "Longitude_GPS"
  Constant9/1 -> Data Type Conversion43/1
  In_GPS/1 -> Bus Selector/1
  Constant14/1 -> Divide4/1
  Constant12/1 -> Divide3/1
  Data Type Conversion43/1 -> Bus Creator/14  "P_code"
  Data Type Conversion/1 -> NOT/1
  Bus Selector/1 -> Data Type Conversion/1  "<GPSModeWord>"
  NOT/1 -> Bus Creator/1  "GPSDataNotValid"

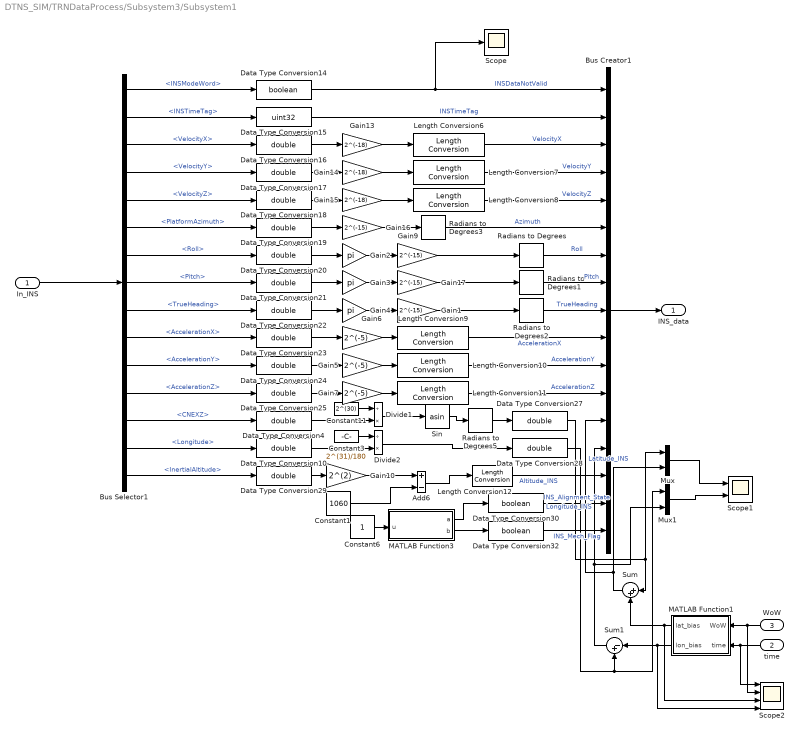
== system DTNS_SIM/TRNDataProcess/Subsystem3/Subsystem1 ==
  In_INS : Inport
  time : Inport  Port=2
  WoW : Inport  Port=3
  Add6 : Sum  Inputs=+-
  Bus Creator1 : BusCreator  Inputs=17  OutDataTypeStr=Bus: TRN_INS  NonVirtualBus=on
      settings: InheritFromInputs=off
  Bus Selector1 : BusSelector  OutputSignals=INSModeWord,INSTimeTag,VelocityX,VelocityY,VelocityZ,PlatformAzimuth,Roll,Pitch,TrueHeading,AccelerationX,AccelerationY,AccelerationZ,CNEXZ,Longitude,InertialAltitude
  Constant1 : Constant  Value=1060
  Constant11 : Constant  Value=2^(30)
  Constant3 : Constant  Value=2^(31)/180
  Constant6 : Constant
  Data Type Conversion{4,10,16..25,27..29} (15 alike) : DataTypeConversion  OutDataTypeStr=double  SaturateOnIntegerOverflow=off  RndMeth=Floor
  Data Type Conversion14 : DataTypeConversion  OutDataTypeStr=boolean  SaturateOnIntegerOverflow=off  RndMeth=Floor
  Data Type Conversion15 : DataTypeConversion  OutDataTypeStr=uint32  SaturateOnIntegerOverflow=off  RndMeth=Floor
  Data Type Conversion30 : DataTypeConversion  OutDataTypeStr=boolean  SaturateOnIntegerOverflow=off  RndMeth=Floor
  Data Type Conversion32 : DataTypeConversion  OutDataTypeStr=boolean  SaturateOnIntegerOverflow=off  RndMeth=Floor
  Divide1 : Product  Inputs=/*
  Divide2 : Product  Inputs=/*
  Gain{1,9,16..17} (4 alike) : Gain  Gain=2^(-15)
  Gain10 : Gain  Gain=2^(2)
  Gain13 : Gain  Gain=2^(-18)
  Gain14 : Gain  Gain=2^(-18)
  Gain15 : Gain  Gain=2^(-18)
  Gain2 : Gain  Gain=pi
  Gain3 : Gain  Gain=pi
  Gain4 : Gain  Gain=pi
  Gain5 : Gain  Gain=2^(-5)
  Gain6 : Gain  Gain=2^(-5)
  Gain7 : Gain  Gain=2^(-5)
  Length Conversion{6..12} (7 alike) : aerolibconvert2/Length Conversion  IU=ft  OU=m
  MATLAB Function1 : MATLAB Function  TreatAsAtomicUnit=on
  MATLAB Function3 : MATLAB Function  TreatAsAtomicUnit=on
  Mux : Mux  Inputs=2
  Mux1 : Mux  Inputs=2
  Radians to Degrees{,1..3,5} (5 alike) : simulink_extras/Transformations/Radians to Degrees
  Scope : Scope
  Scope1 : Scope  NumInputPorts=2
  Scope2 : Scope  NumInputPorts=4
  Sin : Trigonometry  Operator=asin
  Sum : Sum  Inputs=|++
  Sum1 : Sum  Inputs=|-+
  INS_data : Outport
  wires:
  Length Conversion6/1 -> Bus Creator1/3  "VelocityX"
  Constant6/1 -> MATLAB Function3/1(u)
  MATLAB Function3/2(b) -> Data Type Conversion32/1
  Data Type Conversion32/1 -> Bus Creator1/17  "INS_Mech_Flag"
  Data Type Conversion22/1 -> Gain4/1
  Length Conversion9/1 -> Bus Creator1/10  "AccelerationX"
  Data Type Conversion29/1 -> Gain10/1
  Radians to Degrees2/1 -> Bus Creator1/9  "TrueHeading"
  Data Type Conversion16/1 -> Gain13/1
  Data Type Conversion18/1 -> Gain15/1
  Data Type Conversion15/1 -> Bus Creator1/2  "INSTimeTag"
  Bus Selector1/14 -> Data Type Conversion10/1  "<Longitude>"
  Radians to Degrees5/1 -> Data Type Conversion27/1
  Data Type Conversion24/1 -> Gain5/1
  Sin/1 -> Radians to Degrees5/1
  Constant1/1 -> Add6/2
  Gain14/1 -> Length Conversion7/1
  Data Type Conversion14/1 -> Scope/1, Bus Creator1/1  "INSDataNotValid"
  Bus Selector1/5 -> Data Type Conversion18/1  "<VelocityZ>"
  Data Type Conversion25/1 -> Gain7/1
  Divide2/1 -> Data Type Conversion28/1
  MATLAB Function3/1(a) -> Data Type Conversion30/1
  Data Type Conversion19/1 -> Gain16/1
  Bus Selector1/10 -> Data Type Conversion23/1  "<AccelerationX>"
  Data Type Conversion20/1 -> Gain2/1
  Bus Selector1/6 -> Data Type Conversion19/1  "<PlatformAzimuth>"
  Data Type Conversion23/1 -> Gain6/1
  Bus Selector1/7 -> Data Type Conversion20/1  "<Roll>"
  Bus Selector1/2 -> Data Type Conversion15/1  "<INSTimeTag>"
  Bus Selector1/4 -> Data Type Conversion17/1  "<VelocityY>"
  Bus Selector1/3 -> Data Type Conversion16/1  "<VelocityX>"
  Add6/1 -> Length Conversion12/1
  Bus Selector1/15 -> Data Type Conversion29/1  "<InertialAltitude>"
  Bus Selector1/12 -> Data Type Conversion25/1  "<AccelerationZ>"
  Bus Selector1/13 -> Data Type Conversion4/1  "<CNEXZ>"
  Data Type Conversion4/1 -> Divide1/2
  Bus Selector1/9 -> Data Type Conversion22/1  "<TrueHeading>"
  Gain15/1 -> Length Conversion8/1
  Bus Selector1/11 -> Data Type Conversion24/1  "<AccelerationY>"
  Length Conversion12/1 -> Bus Creator1/15  "Altitude_INS"
  Gain6/1 -> Length Conversion9/1
  Data Type Conversion21/1 -> Gain3/1
  Length Conversion8/1 -> Bus Creator1/5  "VelocityZ"
  Data Type Conversion17/1 -> Gain14/1
  Radians to Degrees1/1 -> Bus Creator1/8  "Pitch"
  Length Conversion7/1 -> Bus Creator1/4  "VelocityY"
  Constant3/1 -> Divide2/1
  Gain5/1 -> Length Conversion10/1
  Length Conversion10/1 -> Bus Creator1/11  "AccelerationY"
  Gain7/1 -> Length Conversion11/1
  Radians to Degrees/1 -> Bus Creator1/7  "Roll"
  Divide1/1 -> Sin/1
  Bus Selector1/8 -> Data Type Conversion21/1  "<Pitch>"
  Data Type Conversion10/1 -> Divide2/2
  Data Type Conversion30/1 -> Bus Creator1/16  "INS_Alignment_State"
  Gain10/1 -> Add6/1
  Radians to Degrees3/1 -> Bus Creator1/6  "Azimuth"
  Length Conversion11/1 -> Bus Creator1/12  "AccelerationZ"
  Constant11/1 -> Divide1/1
  Gain16/1 -> Radians to Degrees3/1
  Gain13/1 -> Length Conversion6/1
  Bus Creator1/1 -> INS_data/1
  In_INS/1 -> Bus Selector1/1
  Gain3/1 -> Gain17/1
  Gain4/1 -> Gain1/1
  Gain2/1 -> Gain9/1
  Gain9/1 -> Radians to Degrees/1
  Gain17/1 -> Radians to Degrees1/1
  Gain1/1 -> Radians to Degrees2/1
  Bus Selector1/1 -> Data Type Conversion14/1  "<INSModeWord>"
  Sum/1 -> Bus Creator1/13, Mux/2  "Latitude_INS"
  MATLAB Function1/1(lat_bias) -> Scope2/3, Sum/2
  Sum1/1 -> Mux1/2, Bus Creator1/14  "Longitude_INS"
  MATLAB Function1/2(lon_bias) -> Scope2/4, Sum1/1
  Mux/1 -> Scope1/1
  Mux1/1 -> Scope1/2
  Data Type Conversion27/1 -> Sum/1, Mux/1
  Data Type Conversion28/1 -> Sum1/2, Mux1/1
  WoW/1 -> Scope2/2, MATLAB Function1/1(WoW)
  time/1 -> Scope2/1, MATLAB Function1/2(time)

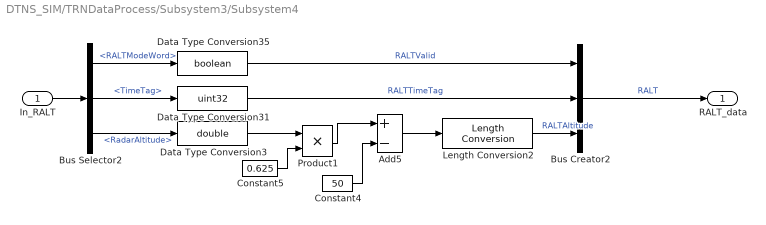
== system DTNS_SIM/TRNDataProcess/Subsystem3/Subsystem4 ==
  In_RALT : Inport
  Add5 : Sum  Inputs=+-
  Bus Creator2 : BusCreator  Inputs=3  OutDataTypeStr=Bus: TRN_RALT  NonVirtualBus=on
      settings: InheritFromInputs=off
  Bus Selector2 : BusSelector  OutputSignals=RALTModeWord,TimeTag,RadarAltitude
  Constant4 : Constant  Value=50
  Constant5 : Constant  Value=0.625
  Data Type Conversion3 : DataTypeConversion  OutDataTypeStr=double  SaturateOnIntegerOverflow=off  RndMeth=Floor
  Data Type Conversion31 : DataTypeConversion  OutDataTypeStr=uint32  SaturateOnIntegerOverflow=off  RndMeth=Floor
  Data Type Conversion35 : DataTypeConversion  OutDataTypeStr=boolean  SaturateOnIntegerOverflow=off  RndMeth=Floor
  Length Conversion2 : aerolibconvert2/Length Conversion  IU=ft  OU=m
  Product1 : Product
  RALT_data : Outport
  wires:
  Length Conversion2/1 -> Bus Creator2/3  "RALTAltitude"
  Constant4/1 -> Add5/2
  Bus Creator2/1 -> RALT_data/1  "RALT"
  In_RALT/1 -> Bus Selector2/1
  Data Type Conversion35/1 -> Bus Creator2/1  "RALTValid"
  Add5/1 -> Length Conversion2/1
  Bus Selector2/3 -> Data Type Conversion3/1  "<RadarAltitude>"
  Data Type Conversion3/1 -> Product1/1
  Product1/1 -> Add5/1
  Constant5/1 -> Product1/2
  Data Type Conversion31/1 -> Bus Creator2/2  "RALTTimeTag"
  Bus Selector2/2 -> Data Type Conversion31/1  "<TimeTag>"
  Bus Selector2/1 -> Data Type Conversion35/1  "<RALTModeWord>"

== matlab function DTNS_SIM/Visualize/calcTerrainRoughness ==
  data: lat input; R output; lon input; hDEM output
function [R, hDEM] = calcTerrainRoughness(lat, lon)

lat2m = 110961.7060516;
lon2m = 89476.51124;

d_Lat = 90/lat2m; d_Lon = 90/lon2m;
d = 90;

hDEM = 0.0;
A=0.0; B=0.0; C=0.0; D=0.0; E=0.0; F=0.0; G=0.0; H=0.0; I=0.0; 

A = coder.ceval('MAPGetTerrainHeight', lat+d_Lat, lon-d_Lon);
B = coder.ceval('MAPGetTerrainHeight', lat+d_Lat, lon);
C = coder.ceval('MAPGetTerrainHeight', lat+d_Lat, lon+d_Lon);
D = coder.ceval('MAPGetTerrainHeight', lat, lon-d_Lon);
E = coder.ceval('MAPGetTerrainHeight', lat, lon);
F = coder.ceval('MAPGetTerrainHeight', lat, lon+d_Lon);
G = coder.ceval('MAPGetTerrainHeight', lat-d_Lat, lon-d_Lon);
H = coder.ceval('MAPGetTerrainHeight', lat-d_Lat, lon);
I = coder.ceval('MAPGetTerrainHeight', lat-d_Lat, lon+d_Lon);

SLP_CR=((C+F+I)-(A+D+G))/(6*d);
SLP_DR=((A+B+C)-(G+H+I))/(6*d);

mean_R=((mean(SLP_CR)-mean(SLP_DR))/2)^2;
std_R=((std(SLP_CR)^2)+(std(SLP_DR)^2))/2;

R=sqrt(mean_R+std_R)*100;

hDEM = E;

end

== matlab function DTNS_SIM/CreateHRInput/ControlHREvent ==
  data: outBus output Bus: HRInput; inBus input Bus: HRInput
function outBus  = ControlHREvent(inBus)
%ControlHREvent
persistent time dt
if isempty(time)
    time = 0.0;
end
if isempty(dt)
    dt = 0.04;
end

ACTIVATED = false;

% Copy
outBus   = inBus;

if ACTIVATED

%     outBus.HRSelected = SET_VALUE(inBus.HRSelected, false, time, 45, 1);

end


time = time + dt;
end


function out = SET_VALUE(in, value, curTime, triggerTime, duration)
out = in;
if (triggerTime <= curTime) && (curTime <= triggerTime+duration)
    out = value;
else
end
end

== matlab function DTNS_SIM/InitNUpdateMapCache/UpdateCache/UpdateCache ==
  data: result output; lat input; lon input; hDEM output
function [result, hDEM] = UpdateCache(lat, lon)
%UpdateCache

% Persistent variables
persistent latPrev lonPrev
if isempty(latPrev)
    latPrev = 0.0;
end
if isempty(lonPrev)
    lonPrev = 0.0;
end

hDEM = 0.0;

% Initialize output
result = int32(1);

if ( abs(lat - latPrev) > 0.05 ) || ( abs(lon - lonPrev) > 0.05)
    result = coder.ceval('UpdateCache', lat, lon);
    hDEM = coder.ceval('MAPGetTerrainHeight', lat, lon);

    if result == 0
        latPrev = lat;
        lonPrev = lon;
    end
else
    
end

== matlab function DTNS_SIM/ControlLOSREvent ==
  data: outBus output Bus: LOSRInput; inBus input Bus: LOSRInput
function outBus  = ControlLOSRSimEvent(inBus)
%ControlAGREvent
persistent time dt
if isempty(time)
    time = 0.0;
end
if isempty(dt)
    dt = 0.04;
end

ACTIVATED = false;

% Copy
outBus   = inBus;

if ACTIVATED

    outBus.LOSRSelected = SET_VALUE(inBus.LOSRSelected, false, time, 35, 1);

end


time = time + dt;
end


function out = SET_VALUE(in, value, curTime, triggerTime, duration)
out = in;
if (triggerTime <= curTime) && (curTime <= triggerTime+duration)
    out = value;
else
end
end

== matlab function DTNS_SIM/InitNUpdateMapCache/InitializeMAP ==
  data: successDTED output; successDVOF output; latDeg input; lonDeg input
function [successDTED, successDVOF] = InitializeMAP(latDeg, lonDeg)
%InitializeMAP

% Persistent variable
persistent firstRun
if isempty(firstRun)
    firstRun = true;
end

% Initialize output
flagDTED = int32(1);
flagDVOF = int32(1);
successDTED = int32(1);
successDVOF = int32(1);
hDEM = 0.0;

if ( IsNear(latDeg, 0) && IsNear(lonDeg, 0) )
    firstRun = true;
    successDTED = int32(1);
    successDVOF = int32(1);
    return
end

if firstRun
    % Path of DTED data
    pathDTED = 'C:\Users\ASCL\Documents\GitHub\DTNS\MAP\MAP_DB';

    % Length of DETD data path
    strLenDTED = int32(strlength(pathDTED));
    
    hDEM = coder.ceval('MAPGetTerrainHeight', latDeg, lonDeg);
    if IsNear(hDEM, -1.0)
        % Call [ InitialMap ] : 맵 폴더 위치 설정
        flagDTED = coder.ceval('InitialMap', pathDTED, strLenDTED );
        successDTED = flagDTED;
        if (~successDTED)
            firstRun = false;
        end
    else
        successDTED = int32(0);
        firstRun = false;       
    end
else
    successDTED = int32(0);
    successDVOF = int32(0);
end

== matlab function DTNS_SIM/CreateHRInput/BallisticComputer ==
  data: TRNOutput input Bus: TRNOutput; selected output; rangeN output; rangeE output; targetElev input; Valid input
function [selected, rangeN, rangeE] = BallisticComputer(TRNOutput, targetElev, Valid)
%BallisticComputer

% Initialize outputs
selected = true;
rangeN = 0.0;
rangeE = 0.0;

x = 0.0;
z = 0.0;


% Rearrange variables
llh = [TRNOutput.TRNEstOfLatitude; ...
    TRNOutput.TRNEstOfLongitude; ...
    TRNOutput.Altitude_INS - TRNOutput.TRNEstOfINSAltitudeErr];

velXYZ = [TRNOutput.TRN_VelocityX; ...
    TRNOutput.TRN_VelocityY; ...
    TRNOutput.TRN_VelocityZ];

attiDeg = [TRNOutput.TRN_Roll; TRNOutput.TRN_Pitch; TRNOutput.TRN_Yaw];

if Valid
    velNED = body2ned(velXYZ, attiDeg);
    V0 = norm(velNED);
    gamma = atan2d(-velNED(3), sqrt(velNED(1)^2+velNED(2)^2));
    z0 = llh(3);
    x0 = 0;
    T = findTime(double(targetElev), z0, V0, gamma);
    if T >= 0

        heading = atan2d(velNED(2), velNED(1));
        [x, z] = bombKinematics(x0, z0, V0, gamma, T);
        selected = true;
        rangeN = x * cosd(heading);
        rangeE = x * sind(heading);
    else
        selected = false;
        rangeN = 0.0;
        rangeE = 0.0;
    end


else
    selected = true;
    rangeN = 0.0;
    rangeE = 0.0;
end

end

%% Internal functions
function [x, z] = bombKinematics(x0, z0, V0, gamma, t)
    
    g = 9.8;
    x = x0 + V0 * cosd(gamma) .* t;
    z = z0 + V0 * sind(gamma) .* t - 0.5 * g * t.^2;
end

function T = findTime(z, z0, V0, gamma)

g = 9.8;

temp = V0^2*(sind(gamma))^2 - 2*g*(z-z0);

if temp < 0
    T = 0;
else
    T = (V0*sind(gamma) + sqrt(V0^2*(sind(gamma))^2 - 2*g*(z-z0) ) ) / g;
end
end

function [state_eb_n, C_b_n] = body2ned(state_eb_b, eulerDeg)
%body2ned
% Compute the transformation from {Body} frame to local {NED} frame
%
% == Inputs =========
% state_eb_b        - states measured w.r.t. {ECEF} and resolved in {Body}
% eulerDeg          - attitude (euler angles roll-pitch-yaw seq.) [deg]
%
% == Outputs ========
% state_eb_n        - xyz-states resolved in {NED}
% C_b_n             - Transformation matirx from {Body} to {NED} (3x3)
% 

state_eb_n  = zeros(3,1);
C_b_n       = zeros(3,3);

% Body to NED
cRol = cosd(eulerDeg(1));
sRol = sind(eulerDeg(1));
cPit = cosd(eulerDeg(2));
sPit = sind(eulerDeg(2));
cYaw = cosd(eulerDeg(3));
sYaw = sind(eulerDeg(3));
% 
% C_n_b   = [              cPit*cYaw,                cPit*sYaw,     -sPit;...
%           sRol*sPit*cYaw-cRol*sYaw, sRol*sPit*sYaw+cRol*cYaw, sRol*cPit;...
%           cRol*sPit*cYaw+sRol*sYaw, cRol*sPit*sYaw-sRol*cYaw, cRol*cPit];

C_b_n   = [ cPit*cYaw, sRol*sPit*cYaw-cRol*sYaw, cRol*sPit*cYaw+sRol*sYaw;...
            cPit*sYaw, sRol*sPit*sYaw+cRol*cYaw, cRol*sPit*sYaw-sRol*cYaw;...
                -sPit,                sRol*cPit,                cRol*cPit];
% C_b_n   = C_n_b';
      
state_eb_n  = C_b_n * state_eb_b;


end
